simulink library "AeroLibrary"  (R2021a)
settings: Solver=VariableStepAuto  StartTime=0.0  StopTime=10.0  RelTol=1e-3
libraries: arduinolib x11, simulink x4, $bdroot x1
settings Model: Creator=42190  LastModifiedBy=42190

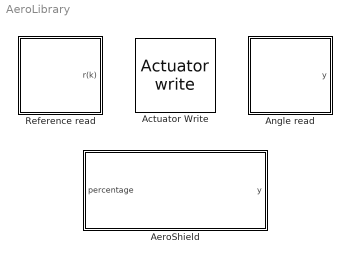
== system AeroLibrary ==
  "Actuator Write " : $bdroot/AeroShield/Actuator write 
  AeroShield : Subsystem
      mask DialogControl DescGroupVar Prompt: AeroShield
      mask DialogControl DescTextVar Prompt: This block represents the AeroShield device. It accepts an input signal for powering the motor in the range of 0-100% and outputs a sensor angle reading in degrees.  Inside this system, you will finde two subsystems. One of them reads the angle of the pendulum and the second one controls the AeroShield actuator.
      mask Display: image('assets\Aero.svg');
  "Angle read " : Subsystem
      mask DialogControl DescGroupVar Prompt: AeroShield angle reading
      mask DialogControl DescTextVar Prompt: Sends commands to AS5600 sensor to read the pendulum angle. Output is in form of 12bit number.
      mask Display: image('assets/Hall.svg');
  Reference read : Subsystem  Variant=on  VariantControlMode=label  LabelModeActiveChoice=Auto  mask{ref=Automatic, model=Others, ButtonRef=off, RefVect=[25 68 35 15 54 75 23 40 80 47], SectLen=200, Ts=0.02}
      mask prompts: ref "Rreference type"; model "Arduino model"; ButtonRef "Use default values"; RefVect "Reference vector:"; SectLen "Section length (number of samples):"; Ts "Sampling period (s):"
      mask init:
      | ref = get_param(gcb,'ref');
      | model = get_param(gcb,'model');
      | 
      | if strcmp(ref,'Manual')
      | if strcmp(model,'Due')
      |     set_param(gcb,'LabelModeActiveChoice', '12bit');
      | elseif strcmp(model,'MKR1000')
      |     set_param(gcb,'LabelModeActiveChoice', '12bit');
      | elseif strcmp(model,'MKR1010')
      |     set_param(gcb,'LabelModeActiveChoice', '12bit');
      | elseif strcmp(model,'MKRZero')
      |     set_param(gcb,'LabelModeActiveChoice', '12bit');
      | elseif strcmp(model,'Nano 33IoT')
      |     set_param(gcb,'LabelModeActiveChoice', '12bit');
      | elseif strcmp(model,'Others') 
      |     set_param(gcb,'LabelModeActiveChoice', '10bit');
      | end
      | end
      | 
      | if strcmp(ref,'Automatic')
      |      set_param(gcb,'LabelModeActiveChoice', 'Auto');
      | end
      mask Help:
      | For basic info, go to https://github.com/gergelytakacs/AutomationShield .
      | For more help, please contact me on my email xtibensky@stuba.sk or ptibensky3@gmail.com.
      mask TypeOptions ref: Manual  | Automatic
      mask Callback ref:
      | ref = get_param(gcb,'ref');
      | 
      | if strcmp(ref(1),'M')
      |     set_param(gcb,'MaskVisibilities',{'on';'on';'off';'off';'off';'off'}),
      | else
      |     set_param(gcb,'MaskVisibilities',{'on';'off';'on';'on';'on';'on'}),
      | end
      mask TypeOptions model: Due | MKR1000 | MKR1010 | MKRZero | Nano 33IoT | Others
      mask Callback model:
      | model = get_param(gcb,'model');
      | if strcmp(model,'Due')
      |     set_param(gcb,'LabelModeActiveChoice', '12bit');
      | elseif strcmp(model,'MKR1000')
      |     set_param(gcb,'LabelModeActiveChoice', '12bit');
      | elseif strcmp(model,'MKR1010')
      |     set_param(gcb,'LabelModeActiveChoice', '12bit');
      | elseif strcmp(model,'MKRZero')
      |     set_param(gcb,'LabelModeActiveChoice', '12bit');
      | elseif strcmp(model,'Nano 33IoT')
      |     set_param(gcb,'LabelModeActiveChoice', '12bit');
      | elseif strcmp(model,'Others')
      |     set_param(gcb,'LabelModeActiveChoice', '10bit');
      | end
      mask Callback ButtonRef:
      | CurrentBlock = gcb;
      | 
      | 
      | set_param(CurrentBlock,'RefVect','[25 68 35 15 54 75 23 40 80 47]');
      | set_param(CurrentBlock,'SectLen','200');
      | set_param(CurrentBlock,'Ts','0.02');
      mask DialogControl DescGroupVar Prompt: AeroShield potentiometer
      mask DialogControl DescTextVar Prompt: Reads potentiometer value from the AeroShield. Returns output in form of percentual value from 0% to 100%.                                                   In dropdown menu, choose your arduino board type.                             In reference type, radio buttons, you can choose between manual or automatic reference trajectory.
      mask Display: image('assets\Potentiometer.svg');

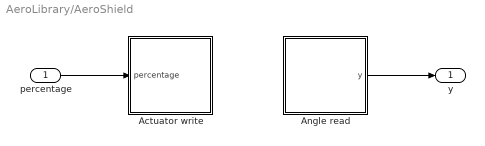
== system AeroLibrary/AeroShield ==
  percentage : Inport
  "Actuator write " : Subsystem
      mask DialogControl DescGroupVar Prompt: AeroShield actuator
      mask DialogControl DescTextVar Prompt: Sets speed level to the dc motor at the end of the AeroShield pendulum. Expects input in form of percentual value from 0% to 100%.
      mask Display: image('assets/Fan.svg');
  "Angle read " : Subsystem
      mask DialogControl DescGroupVar Prompt: AeroShield angle reading
      mask DialogControl DescTextVar Prompt: Sends commands to AS5600 sensor to read the pendulum angle. Output is in form of 12bit number.
      mask Display: image('assets/angle.svg');
  y : Outport
  wires:
  percentage/1 -> "Actuator write "/1(percentage)
  "Angle read "/1(y) -> y/1

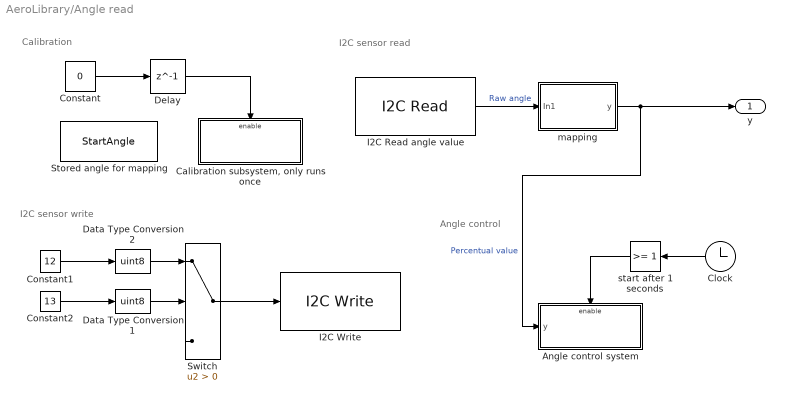
== system AeroLibrary/Angle read  ==
  note: Angle control
  note: I2C sensor read
  note: I2C sensor write
  note: Calibration
  Angle control system : Subsystem  TreatAsAtomicUnit=on
  "Calibration subsystem, only runs once" : Subsystem  TreatAsAtomicUnit=on
  Clock : Clock
      settings: Decimation=100
  Constant : Constant  Value=0
  Constant1 : Constant  Value=12
  Constant2 : Constant  Value=13
  Data Type Conversion1 : DataTypeConversion  OutDataTypeStr=uint8
  Data Type Conversion2 : DataTypeConversion  OutDataTypeStr=uint8
  Delay : Delay  DelayLength=1  InitialCondition=1
  I2C Read angle value : arduinolib/I2C Read  I2CModule=0  Mode=Master  SlaveAddress=uint8(hex2dec('36'))  SlaveByteOrder=BigEndian  Direction=Receiver  RegisterAddressMode=off  RegisterAddress=uint8(hex2dec('36'))  SlaveDataType=uint16  DataLength=1  NoAck=off  RepeatedStart=off  OutputStatus=off  blockPlatform=ARDUINO  SampleTime=-1
      settings: SourceProductBaseCode=ARDUINO
  I2C Write : arduinolib/I2C Write  I2CModule=0  Mode=Master  SlaveAddress=uint8(hex2dec('36'))  SlaveByteOrder=BigEndian  Direction=Transmitter  RegisterAddressMode=off  RegisterAddress=uint8(hex2dec('0c'))  SlaveDataType=uint8  DataLength=1  NoAck=off  RepeatedStart=off  OutputStatus=off  blockPlatform=ARDUINO
      settings: SourceProductBaseCode=ARDUINO
  Stored angle for mapping : DataStoreMemory  DataStoreName=StartAngle  ReadBeforeWriteMsg=warning  WriteAfterWriteMsg=warning  WriteAfterReadMsg=warning  ShowAdditionalParam=off
  Switch : Switch  Criteria=u2 > Threshold
  mapping : Subsystem
  start after 1 seconds : simulink/Logic and Bit Operations/Compare To Constant  relop=>=  const=1  OutDataTypeStr=boolean
  y : Outport
  wires:
  start after 1 seconds/1 -> Angle control system/Enable
  Clock/1 -> start after 1 seconds/1
  mapping/1(y) -> y/1, Angle control system/1(y)  "Percentual value"
  Constant/1 -> Delay/1
  Delay/1 -> "Calibration subsystem, only runs once"/Enable
  I2C Read angle value/1 -> mapping/1(In1)  "Raw angle"
  ? -> Switch/3
  Constant1/1 -> Data Type Conversion2/1
  Constant2/1 -> Data Type Conversion1/1
  Switch/1 -> I2C Write/1
  Data Type Conversion2/1 -> Switch/1
  Data Type Conversion1/1 -> Switch/2

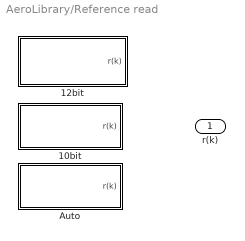
== system AeroLibrary/Reference read ==
  10bit : Subsystem  VariantControl=10bit
  12bit : Subsystem  VariantControl=12bit
  Auto : Subsystem  VariantControl=Auto
  r(k) : Outport

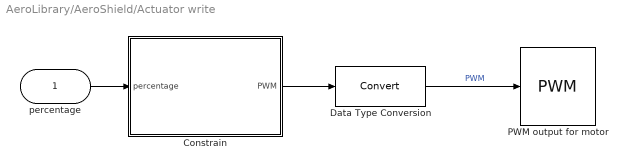
== system AeroLibrary/AeroShield/Actuator write  ==
  percentage : Inport
  Constrain : MATLAB Function  TreatAsAtomicUnit=on
  Data Type Conversion : DataTypeConversion
  "PWM output for motor " : arduinolib/PWM  pinNumber=5  frequencyType=Default  desiredFrequency=490.2  achievableFrequency=490.2
  wires:
  percentage/1 -> Constrain/1(percentage)
  Data Type Conversion/1 -> "PWM output for motor "/1  "PWM"
  Constrain/1(PWM) -> Data Type Conversion/1

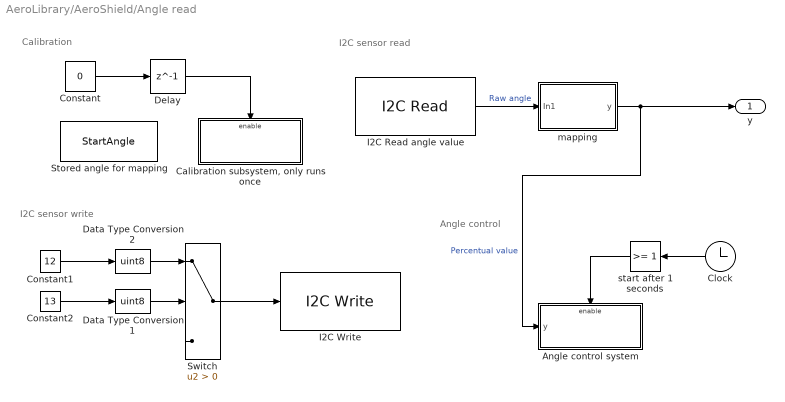
== system AeroLibrary/AeroShield/Angle read  ==
  note: Calibration
  note: I2C sensor write
  note: I2C sensor read
  note: Angle control
  Angle control system : Subsystem  TreatAsAtomicUnit=on
  "Calibration subsystem, only runs once" : Subsystem  TreatAsAtomicUnit=on
  Clock : Clock
      settings: Decimation=100
  Constant : Constant  Value=0
  Constant1 : Constant  Value=12
  Constant2 : Constant  Value=13
  Data Type Conversion1 : DataTypeConversion  OutDataTypeStr=uint8
  Data Type Conversion2 : DataTypeConversion  OutDataTypeStr=uint8
  Delay : Delay  DelayLength=1  InitialCondition=1
  I2C Read angle value : arduinolib/I2C Read  I2CModule=0  Mode=Master  SlaveAddress=uint8(hex2dec('36'))  SlaveByteOrder=BigEndian  Direction=Receiver  RegisterAddressMode=off  RegisterAddress=uint8(hex2dec('36'))  SlaveDataType=uint16  DataLength=1  NoAck=off  RepeatedStart=off  OutputStatus=off  blockPlatform=ARDUINO  SampleTime=-1
      settings: SourceProductBaseCode=ARDUINO
  I2C Write : arduinolib/I2C Write  I2CModule=0  Mode=Master  SlaveAddress=uint8(hex2dec('36'))  SlaveByteOrder=BigEndian  Direction=Transmitter  RegisterAddressMode=off  RegisterAddress=uint8(hex2dec('0c'))  SlaveDataType=uint8  DataLength=1  NoAck=off  RepeatedStart=off  OutputStatus=off  blockPlatform=ARDUINO
      settings: SourceProductBaseCode=ARDUINO
  Stored angle for mapping : DataStoreMemory  DataStoreName=StartAngle  ReadBeforeWriteMsg=warning  WriteAfterWriteMsg=warning  WriteAfterReadMsg=warning  ShowAdditionalParam=off
  Switch : Switch  Criteria=u2 > Threshold
  mapping : Subsystem
  start after 1 seconds : simulink/Logic and Bit Operations/Compare To Constant  relop=>=  const=1  OutDataTypeStr=boolean
  y : Outport
  wires:
  Data Type Conversion1/1 -> Switch/2
  Data Type Conversion2/1 -> Switch/1
  Switch/1 -> I2C Write/1
  Constant2/1 -> Data Type Conversion1/1
  Constant1/1 -> Data Type Conversion2/1
  ? -> Switch/3
  I2C Read angle value/1 -> mapping/1(In1)  "Raw angle"
  Delay/1 -> "Calibration subsystem, only runs once"/Enable
  Constant/1 -> Delay/1
  mapping/1(y) -> Angle control system/1(y), y/1  "Percentual value"
  Clock/1 -> start after 1 seconds/1
  start after 1 seconds/1 -> Angle control system/Enable

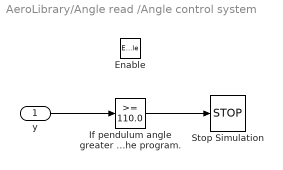
== system AeroLibrary/Angle read /Angle control system ==
  y : Inport
  Enable : EnablePort
  "If pendulum angle greater than 110°, stop the program." : simulink/Logic and Bit Operations/Compare To Constant  relop=>=  const=110.0  OutDataTypeStr=boolean
  Stop Simulation : Stop
  wires:
  "If pendulum angle greater than 110°, stop the program."/1 -> Stop Simulation/1
  y/1 -> "If pendulum angle greater than 110°, stop the program."/1

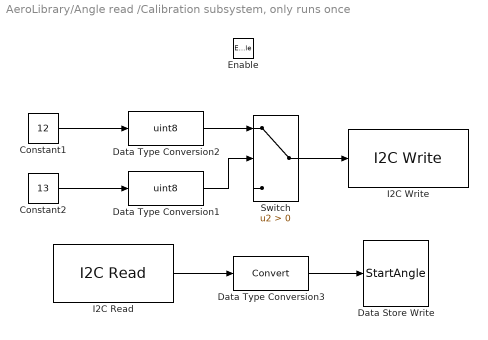
== system AeroLibrary/Angle read /Calibration subsystem, only runs once ==
  Enable : EnablePort
  Constant1 : Constant  Value=12
  Constant2 : Constant  Value=13
  Data Store Write : DataStoreWrite  DataStoreName=StartAngle  IndexOptions=Index vector (dialog)  Indices=1  OutputSizes=1
  Data Type Conversion1 : DataTypeConversion  OutDataTypeStr=uint8
  Data Type Conversion2 : DataTypeConversion  OutDataTypeStr=uint8
  Data Type Conversion3 : DataTypeConversion
  I2C Read : arduinolib/I2C Read  I2CModule=0  Mode=Master  SlaveAddress=uint8(hex2dec('36'))  SlaveByteOrder=BigEndian  Direction=Receiver  RegisterAddressMode=off  RegisterAddress=uint8(hex2dec('36'))  SlaveDataType=uint16  DataLength=1  NoAck=off  RepeatedStart=off  OutputStatus=off  blockPlatform=ARDUINO  SampleTime=-1
      settings: SourceProductBaseCode=ARDUINO
  I2C Write : arduinolib/I2C Write  I2CModule=0  Mode=Master  SlaveAddress=uint8(hex2dec('36'))  SlaveByteOrder=BigEndian  Direction=Transmitter  RegisterAddressMode=off  RegisterAddress=uint8(hex2dec('0c'))  SlaveDataType=uint8  DataLength=1  NoAck=off  RepeatedStart=off  OutputStatus=off  blockPlatform=ARDUINO
      settings: SourceProductBaseCode=ARDUINO
  Switch : Switch  Criteria=u2 > Threshold
  wires:
  Constant2/1 -> Data Type Conversion1/1
  I2C Read/1 -> Data Type Conversion3/1
  Data Type Conversion2/1 -> Switch/1
  Data Type Conversion1/1 -> Switch/2
  Constant1/1 -> Data Type Conversion2/1
  Switch/1 -> I2C Write/1
  Data Type Conversion3/1 -> Data Store Write/1

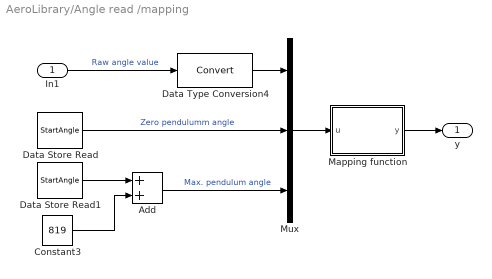
== system AeroLibrary/Angle read /mapping ==
  In1 : Inport
  Add : Sum
  Constant3 : Constant  Value=819
  Data Store Read : DataStoreRead  DataStoreName=StartAngle  IndexOptions=Index vector (dialog)  Indices=1  OutputSizes=1
  Data Store Read1 : DataStoreRead  DataStoreName=StartAngle  IndexOptions=Index vector (dialog)  Indices=1  OutputSizes=1
  Data Type Conversion4 : DataTypeConversion
  Mapping function : MATLAB Function  TreatAsAtomicUnit=on
  Mux : Mux  Inputs=3
  y : Outport
  wires:
  Constant3/1 -> Add/2
  Data Store Read/1 -> Mux/2  "Zero pendulumm angle"
  In1/1 -> Data Type Conversion4/1  "Raw angle value"
  Add/1 -> Mux/3  "Max. pendulum angle"
  Mapping function/1(y) -> y/1
  Data Store Read1/1 -> Add/1
  Mux/1 -> Mapping function/1(u)
  Data Type Conversion4/1 -> Mux/1

== system AeroLibrary/Reference read/10bit ==
  Analog Input : arduinolib/Analog Input  pinNumber=3  ReadResultsOnly=off  ConversionTriggerSource=Software  ExternalTriggerType=uint32( 0 )  OutputDataType=uint16  EnableConversionCompleteNotify=off  EnableOuputStatus=off  SampleTime=-1  blockPlatform=arduino
  Gain1 : Gain  Gain=1/10.24
  r(k) : Outport
  wires:
  Analog Input/1 -> Gain1/1  "Analog potentiometer value"
  Gain1/1 -> r(k)/1  "Percentual value"

== system AeroLibrary/Reference read/12bit ==
  Analog Input : arduinolib/Analog Input  pinNumber=3  ReadResultsOnly=off  ConversionTriggerSource=Software  ExternalTriggerType=uint32( 0 )  OutputDataType=uint16  EnableConversionCompleteNotify=off  EnableOuputStatus=off  SampleTime=-1  blockPlatform=arduino
  Gain1 : Gain  Gain=1/40.95
  r(k) : Outport
  wires:
  Analog Input/1 -> Gain1/1  "Analog potentiometer value"
  Gain1/1 -> r(k)/1  "Percentage value"

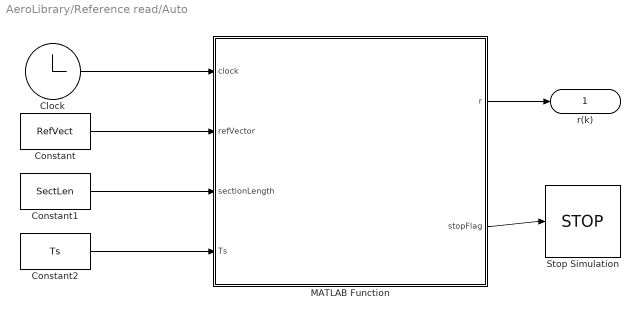
== system AeroLibrary/Reference read/Auto ==
  Clock : Clock
  Constant : Constant  Value=RefVect  SampleTime=Ts
  Constant1 : Constant  Value=SectLen  SampleTime=Ts
  Constant2 : Constant  Value=Ts  SampleTime=Ts
  MATLAB Function : MATLAB Function  TreatAsAtomicUnit=on
  Stop Simulation : Stop
  r(k) : Outport
  wires:
  MATLAB Function/1(r) -> r(k)/1
  MATLAB Function/2(stopFlag) -> Stop Simulation/1
  Clock/1 -> MATLAB Function/1(clock)
  Constant/1 -> MATLAB Function/2(refVector)
  Constant1/1 -> MATLAB Function/3(sectionLength)
  Constant2/1 -> MATLAB Function/4(Ts)

== system AeroLibrary/AeroShield/Angle read /Angle control system ==
  y : Inport
  Enable : EnablePort
  "If pendulum angle greater than 110°, stop the program." : simulink/Logic and Bit Operations/Compare To Constant  relop=>=  const=110.0  OutDataTypeStr=boolean
  Stop Simulation : Stop
  wires:
  y/1 -> "If pendulum angle greater than 110°, stop the program."/1
  "If pendulum angle greater than 110°, stop the program."/1 -> Stop Simulation/1

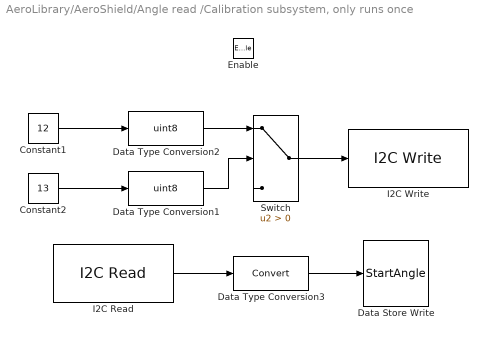
== system AeroLibrary/AeroShield/Angle read /Calibration subsystem, only runs once ==
  Enable : EnablePort
  Constant1 : Constant  Value=12
  Constant2 : Constant  Value=13
  Data Store Write : DataStoreWrite  DataStoreName=StartAngle  IndexOptions=Index vector (dialog)  Indices=1  OutputSizes=1
  Data Type Conversion1 : DataTypeConversion  OutDataTypeStr=uint8
  Data Type Conversion2 : DataTypeConversion  OutDataTypeStr=uint8
  Data Type Conversion3 : DataTypeConversion
  I2C Read : arduinolib/I2C Read  I2CModule=0  Mode=Master  SlaveAddress=uint8(hex2dec('36'))  SlaveByteOrder=BigEndian  Direction=Receiver  RegisterAddressMode=off  RegisterAddress=uint8(hex2dec('36'))  SlaveDataType=uint16  DataLength=1  NoAck=off  RepeatedStart=off  OutputStatus=off  blockPlatform=ARDUINO  SampleTime=-1
      settings: SourceProductBaseCode=ARDUINO
  I2C Write : arduinolib/I2C Write  I2CModule=0  Mode=Master  SlaveAddress=uint8(hex2dec('36'))  SlaveByteOrder=BigEndian  Direction=Transmitter  RegisterAddressMode=off  RegisterAddress=uint8(hex2dec('0c'))  SlaveDataType=uint8  DataLength=1  NoAck=off  RepeatedStart=off  OutputStatus=off  blockPlatform=ARDUINO
      settings: SourceProductBaseCode=ARDUINO
  Switch : Switch  Criteria=u2 > Threshold
  wires:
  Data Type Conversion3/1 -> Data Store Write/1
  Switch/1 -> I2C Write/1
  Constant1/1 -> Data Type Conversion2/1
  Data Type Conversion1/1 -> Switch/2
  Data Type Conversion2/1 -> Switch/1
  I2C Read/1 -> Data Type Conversion3/1
  Constant2/1 -> Data Type Conversion1/1

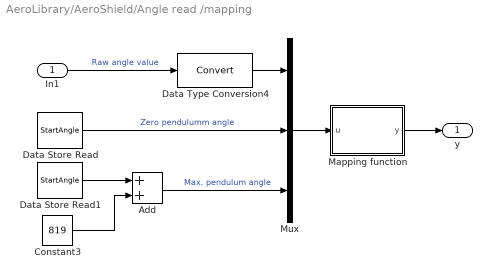
== system AeroLibrary/AeroShield/Angle read /mapping ==
  In1 : Inport
  Add : Sum
  Constant3 : Constant  Value=819
  Data Store Read : DataStoreRead  DataStoreName=StartAngle  IndexOptions=Index vector (dialog)  Indices=1  OutputSizes=1
  Data Store Read1 : DataStoreRead  DataStoreName=StartAngle  IndexOptions=Index vector (dialog)  Indices=1  OutputSizes=1
  Data Type Conversion4 : DataTypeConversion
  Mapping function : MATLAB Function  TreatAsAtomicUnit=on
  Mux : Mux  Inputs=3
  y : Outport
  wires:
  Data Type Conversion4/1 -> Mux/1
  Mux/1 -> Mapping function/1(u)
  Data Store Read1/1 -> Add/1
  Mapping function/1(y) -> y/1
  Add/1 -> Mux/3  "Max. pendulum angle"
  In1/1 -> Data Type Conversion4/1  "Raw angle value"
  Data Store Read/1 -> Mux/2  "Zero pendulumm angle"
  Constant3/1 -> Add/2

== matlab function AeroLibrary/Angle read /mapping/Mapping function ==
  data: u input; y output
function y = fcn(u)
angMin=0;
angMax=72;
y = ((u(1) - u(2)) * (angMax - angMin)) / (u(3) - u(2)) + angMin ;

== matlab function AeroLibrary/AeroShield/Actuator write /Constrain ==
  data: percentage input; PWM output
function PWM = fcn(percentage)

PWM = constrain((percentage * 2.55), 0, 255);

end

== matlab function AeroLibrary/AeroShield/Angle read /mapping/Mapping function ==
  data: u input; y output
function y = fcn(u)
angMin=0;
angMax=72;
y = ((u(1) - u(2)) * (angMax - angMin)) / (u(3) - u(2)) + angMin ;

== matlab function AeroLibrary/Reference read/Auto/MATLAB Function ==
  data: clock input; r output; refVector input; sectionLength input; Ts input; stopFlag output
function [r, stopFlag] = fcn(clock, refVector, sectionLength, Ts)

persistent counter;

pauseTime = 2;

if isempty(counter)
    counter = 1;
end

if clock > pauseTime
    RefLength = length(refVector);
    SectionDuration = sectionLength * Ts;
    if (clock - pauseTime) <= (SectionDuration * counter)
        r = refVector(counter);
        stopFlag = 0;
    else
        counter = counter + 1;
        if counter <= RefLength
            r = refVector(counter);
            stopFlag = 0;
        else
            r = refVector(counter-1);
            stopFlag = 1; 
        end
    end
else
    r = refVector(1);
    stopFlag = 0;
end

end
